simulink model "model_wahadla_lepkie"  (R2023a)
settings: Solver=ode45  StartTime=0.0  StopTime=end_time  FixedStep=dt  MaxStep=0.001  RelTol=1e-3
values from neighbouring files (symbols this model uses):
  IC = [0;pi;0;0]    [system_id_2.m]
settings Model: SimulationMode=accelerator  Creator=Adam  LastModifiedBy=Adam
settings SolverCC: AlgebraicLoopSolver=TrustRegion
settings DataIOCC: ExternalInput=ind  LoadExternalInput=on  SignalLogging=off  DSMLogging=off  OutputSaveName=out  ReturnWorkspaceOutputsName=sout
settings OptimizationCC: SimCompilerOptimization=on  AccelVerboseBuild=on
settings DebuggingCC: AlgebraicLoopMsg=none  UnconnectedInputMsg=warning  UnconnectedOutputMsg=warning  UnconnectedLineMsg=warning
settings ModelReferenceCC: EnableRefExpFcnMdlSchedulingChecks=on
settings RTWCC: DLArmComputeVersion=19.05

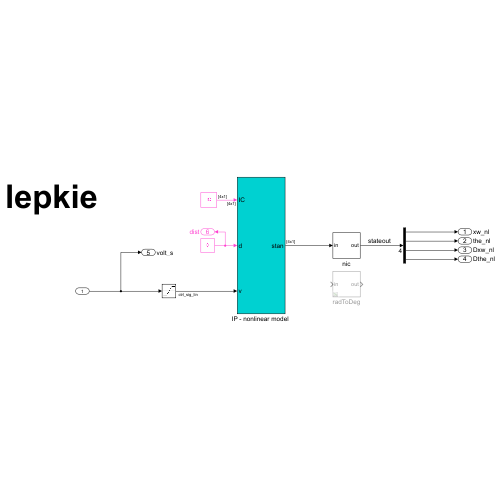
[thumbnail: Simulink's stored preview of the top-level diagram]
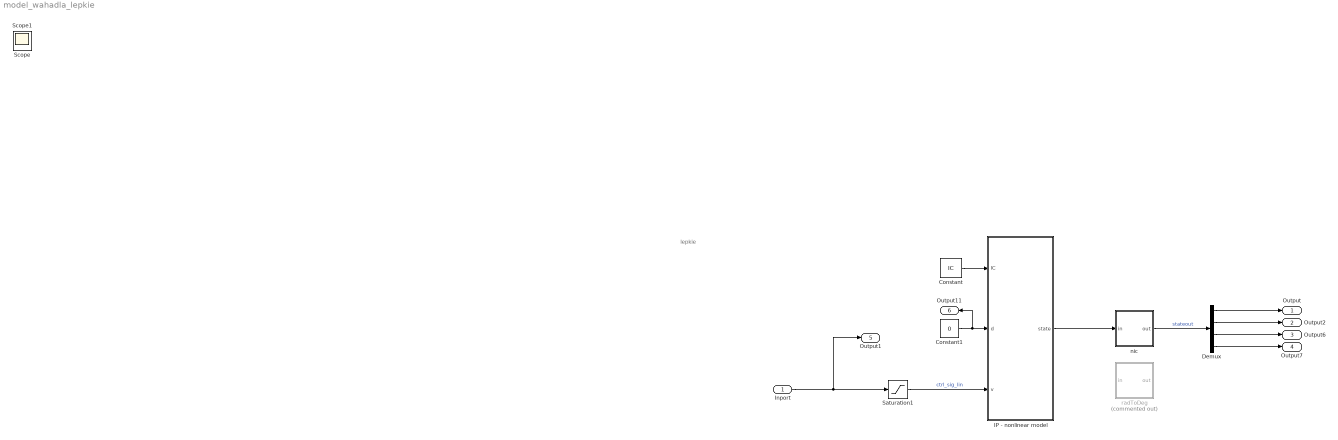
== system model_wahadla_lepkie ==
  note: lepkie
  Inport : Inport
  Constant : Constant  Value=IC  VectorParams1D=off
  Constant1 : Constant  Value=0
  Demux : Demux
  "IP - nonlinear model " : Subsystem  Description=Nonlinear model of inverted pendulum
      mask Display:
      | port_label('output', 1, 'stan');
      | port_label('input', 1, 'IC');
      | port_label('input', 2, 'd');
      | port_label('input', 3, 'v');
  Saturation1 : Saturate  UpperLimit=12  LowerLimit=-12
  nic : Subsystem
  radToDeg : Subsystem  Commented=on
  Output : Outport  SignalName=xw_nl
  Output2 : Outport  Port=2  SignalName=the_nl
  Output6 : Outport  Port=3  SignalName=Dxw_nl
  Output7 : Outport  Port=4  SignalName=Dthe_nl
  Output1 : Outport  Port=5  SignalName=volt_s
  Output11 : Outport  Port=6  SignalName=dist
  Scope : Scope
  Scope1 : Scope
  wires:
  "IP - nonlinear model "/1(state) -> nic/1(in)
  Constant/1 -> "IP - nonlinear model "/1(IC)
  Constant1/1 -> "IP - nonlinear model "/2(d), Output11/1
  nic/1(out) -> Demux/1  "stateout"
  Demux/1 -> Output/1
  Demux/2 -> Output2/1
  Demux/3 -> Output6/1
  Demux/4 -> Output7/1
  Inport/1 -> Saturation1/1, Output1/1
  Saturation1/1 -> "IP - nonlinear model "/3(v)  "ctrl_sig_lin"

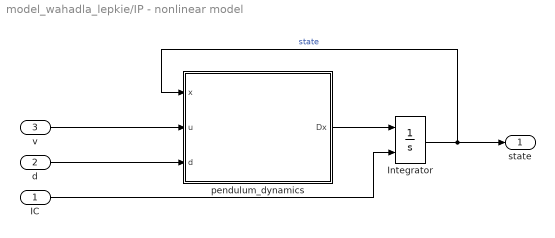
== system model_wahadla_lepkie/IP - nonlinear model  ==
  IC : Inport
  d : Inport  Port=2
  v : Inport  Port=3
  Integrator : Integrator  InitialConditionSource=external
  pendulum_dynamics : MATLAB Function  TreatAsAtomicUnit=on
  state : Outport
  wires:
  Integrator/1 -> state/1, pendulum_dynamics/1(x)  "state"
  v/1 -> pendulum_dynamics/2(u)
  pendulum_dynamics/1(Dx) -> Integrator/1
  IC/1 -> Integrator/2
  d/1 -> pendulum_dynamics/3(d)

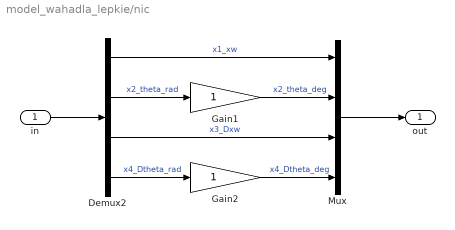
== system model_wahadla_lepkie/nic ==
  in : Inport
  Demux2 : Demux
  Gain1 : Gain
  Gain2 : Gain
  Mux : Mux
  out : Outport
  wires:
  Demux2/1 -> Mux/1  "x1_xw"
  Gain1/1 -> Mux/2  "x2_theta_deg"
  Gain2/1 -> Mux/4  "x4_Dtheta_deg"
  Demux2/2 -> Gain1/1  "x2_theta_rad"
  in/1 -> Demux2/1
  Demux2/3 -> Mux/3  "x3_Dxw"
  Demux2/4 -> Gain2/1  "x4_Dtheta_rad"
  Mux/1 -> out/1

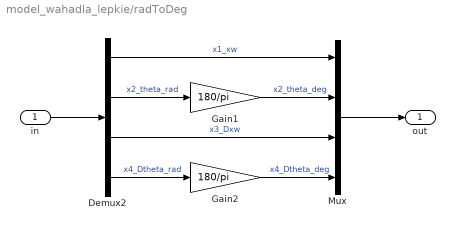
== system model_wahadla_lepkie/radToDeg ==
  in : Inport
  Demux2 : Demux
  Gain1 : Gain  Gain=180/pi
  Gain2 : Gain  Gain=180/pi
  Mux : Mux
  out : Outport
  wires:
  Demux2/1 -> Mux/1  "x1_xw"
  Gain1/1 -> Mux/2  "x2_theta_deg"
  Gain2/1 -> Mux/4  "x4_Dtheta_deg"
  Demux2/2 -> Gain1/1  "x2_theta_rad"
  in/1 -> Demux2/1
  Demux2/3 -> Mux/3  "x3_Dxw"
  Demux2/4 -> Gain2/1  "x4_Dtheta_rad"
  Mux/1 -> out/1

== matlab function model_wahadla_lepkie/IP - nonlinear model /pendulum_dynamics ==
  data: x input; u input; d input; Dx output; params_lepkie parameter
function Dx = dynamika_wahadla(x, u, d, params_lepkie)
% x : stan
% u : input - napięcie
%
% params scope: "parameters"
%

% State, function input: x = [x Dx theta Dtheta]'
x1 = x(1);
x2 = x(2); 
x3 = x(3);
x4 = x(4);

params_lepkie = num2cell(params_lepkie);
% [M, mc, mp, Lp, Lc, g, b, gamma, mr, Mt, L, Jcm, Jt, alpha, beta] = params_lepkie{:};
[M, mp, mc, Lp, B, gamma_vis, alpha_dcm] = params_lepkie{:};

g = 9.8145;
Lc = 2*Lp;
mr = mc + mp;
Mt = mr + M;
L = (Lc*mc + Lp*mp) / mr;
Jcm = 1/12*mp*Lp^2;
Jt = Jcm + mr*L^2;

% Equations for pendulum dynamics
% Ff = b*x3;
% Fi = alpha_dcm*u - beta_dcm*x3;
% A = d*cos(x2) - Ff + L*mr*x4^2*sin(x2) + Fi;
A = d*cos(x2) + L*mr*x4^2*sin(x2) + alpha_dcm*u - B*x3;
B = d*Lc + L*g*mr*sin(x2) - gamma_vis*x4;
DEN = Jt*Mt - (L*mr*cos(x2))^2;

ddt_x1 = x3;
ddt_x2 = x4;
ddt_x3 = (Jt*A - L*mr*cos(x2)*B) / DEN;
ddt_x4 = (Mt*B - L*mr*cos(x2)*A) / DEN;

% output (wektor kolumnowy)
Dx = [ddt_x1 ddt_x2 ddt_x3 ddt_x4]';
end
